simulink model "MPC"  (R2018b)
settings: Solver=VariableStepAuto  StartTime=0.0  StopTime=5  RelTol=1e-3
libraries: mpclib x2
settings Model: Creator=dongdaming  LastModifiedBy=dongdaming

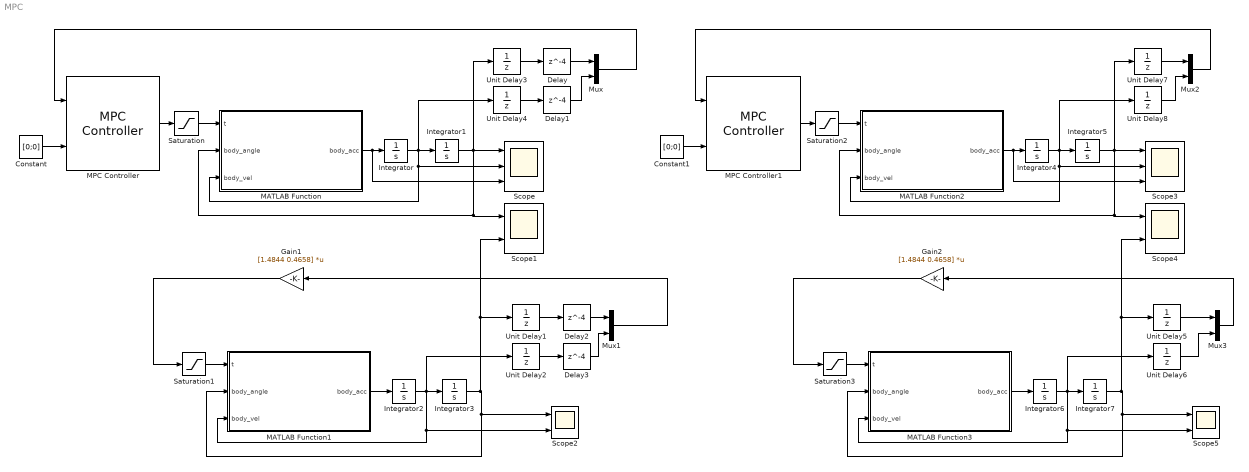
== system MPC ==
  Constant : Constant  Value=[0;0]
  Constant1 : Constant  Value=[0;0]
  Delay{,1..3} (4 alike) : Delay  DelayLength=4
  Gain1 : Gain  Gain=[1.4844 0.4658]  Multiplication=Matrix(K*u)
  Gain2 : Gain  Gain=[1.4844 0.4658]  Multiplication=Matrix(K*u)
  Integrator{,2,4,6} (4 alike) : Integrator
  Integrator1 : Integrator  InitialCondition=pi/3  UpperSaturationLimit=pi  LowerSaturationLimit=-pi
  Integrator3 : Integrator  InitialCondition=pi/3  LimitOutput=on  UpperSaturationLimit=pi  LowerSaturationLimit=-pi
  Integrator5 : Integrator  InitialCondition=pi/3  UpperSaturationLimit=pi  LowerSaturationLimit=-pi
  Integrator7 : Integrator  InitialCondition=pi/3  LimitOutput=on  UpperSaturationLimit=pi  LowerSaturationLimit=-pi
  MATLAB Function : MATLAB Function  TreatAsAtomicUnit=on
  MATLAB Function1 : MATLAB Function  TreatAsAtomicUnit=on
  MATLAB Function2 : MATLAB Function  TreatAsAtomicUnit=on
  MATLAB Function3 : MATLAB Function  TreatAsAtomicUnit=on
  MPC Controller : mpclib/MPC Controller  SCDEnableBlockLinearizationSpecification=on  mpcobj=mpc1  is_multiple=0  enable_value=0  return_u0=off  updateMPCinCallerWorkspace=on  md_inport=off  mv_inport=off  return_cost=off  return_mvseq=off  return_qpstatus=off  return_xseq=off  return_state=off  return_ovseq=off  state_inport=off  umin_inport=off  umax_inport=off  ymin_inport=off  ymax_inport=off  cc_inport=off  ywt_inport=off  uwt_inport=off  duwt_inport=off  rhoeps_inport=off  uref_inport=off  n_ts=0.002  n_p=20  n_mv=1  n_md=0  n_ud=0  n_mo=2  n_uo=0  BlockDataType=double  SampleTimeInherited=off  switch_inport=off
  MPC Controller1 : mpclib/MPC Controller  SCDEnableBlockLinearizationSpecification=on  mpcobj=mpc1  is_multiple=0  enable_value=0  return_u0=off  updateMPCinCallerWorkspace=on  md_inport=off  mv_inport=off  return_cost=off  return_mvseq=off  return_qpstatus=off  return_xseq=off  return_state=off  return_ovseq=off  state_inport=off  umin_inport=off  umax_inport=off  ymin_inport=off  ymax_inport=off  cc_inport=off  ywt_inport=off  uwt_inport=off  duwt_inport=off  rhoeps_inport=off  uref_inport=off  n_ts=0.002  n_p=20  n_mv=1  n_md=0  n_ud=0  n_mo=2  n_uo=0  BlockDataType=double  SampleTimeInherited=off  switch_inport=off
  Mux{,1..3} (4 alike) : Mux  Inputs=2
  Saturation{,1..3} (4 alike) : Saturate  UpperLimit=1.4  LowerLimit=-1.4
  Scope : Scope  NumInputPorts=3
  Scope{1..2,4..5} (4 alike) : Scope  NumInputPorts=2
  Scope3 : Scope  NumInputPorts=3
  Unit Delay{1,3,5,7} (4 alike) : UnitDelay  SampleTime=0.002
  Unit Delay{2,4,6,8} (4 alike) : UnitDelay  InitialCondition=pi/3  SampleTime=0.002
  wires:
  Integrator/1 -> Unit Delay4/1, MATLAB Function/3(body_vel), Scope/2, Integrator1/1
  Integrator1/1 -> Unit Delay3/1, Scope1/1, MATLAB Function/2(body_angle), Scope/1
  Constant/1 -> MPC Controller/2
  Mux/1 -> MPC Controller/1
  MATLAB Function/1(body_acc) -> Scope/3, Integrator/1
  Saturation/1 -> MATLAB Function/1(t)
  MPC Controller/1 -> Saturation/1
  Saturation1/1 -> MATLAB Function1/1(t)
  MATLAB Function1/1(body_acc) -> Integrator2/1
  Integrator3/1 -> Scope1/2, Unit Delay1/1, MATLAB Function1/2(body_angle), Scope2/1
  Integrator2/1 -> Unit Delay2/1, Integrator3/1, Scope2/2, MATLAB Function1/3(body_vel)
  Gain1/1 -> Saturation1/1
  Mux1/1 -> Gain1/1
  Unit Delay3/1 -> Delay/1
  Delay/1 -> Mux/1
  Unit Delay4/1 -> Delay1/1
  Delay1/1 -> Mux/2
  Unit Delay1/1 -> Delay2/1
  Delay2/1 -> Mux1/1
  Unit Delay2/1 -> Delay3/1
  Delay3/1 -> Mux1/2
  Unit Delay6/1 -> Mux3/2
  Unit Delay5/1 -> Mux3/1
  Unit Delay8/1 -> Mux2/2
  Unit Delay7/1 -> Mux2/1
  Mux3/1 -> Gain2/1
  Gain2/1 -> Saturation3/1
  Integrator6/1 -> MATLAB Function3/3(body_vel), Scope5/2, Integrator7/1, Unit Delay6/1
  Integrator7/1 -> Scope5/1, MATLAB Function3/2(body_angle), Unit Delay5/1, Scope4/2
  MATLAB Function3/1(body_acc) -> Integrator6/1
  Saturation3/1 -> MATLAB Function3/1(t)
  MPC Controller1/1 -> Saturation2/1
  Saturation2/1 -> MATLAB Function2/1(t)
  MATLAB Function2/1(body_acc) -> Integrator4/1, Scope3/3
  Mux2/1 -> MPC Controller1/1
  Constant1/1 -> MPC Controller1/2
  Integrator5/1 -> Scope3/1, MATLAB Function2/2(body_angle), Scope4/1, Unit Delay7/1
  Integrator4/1 -> Integrator5/1, Scope3/2, MATLAB Function2/3(body_vel), Unit Delay8/1

== matlab function MPC/MATLAB Function1 ==
  data: t input; body_acc output; body_angle input; body_vel input
function body_acc = fcn(t,body_angle,body_vel)
body_acc=(+1429.48*sin(body_angle)-1215.55*t-2083.85*t*cos(body_angle)-3.87597*sin(2*body_angle)*body_vel^2)/(2.91931+cos(body_angle)^2+8.75194*sin(body_angle)^2);

== matlab function MPC/MATLAB Function ==
  data: t input; body_acc output; body_angle input; body_vel input
function body_acc = fcn(t,body_angle,body_vel)
body_acc=(+1429.48*sin(body_angle)-1215.55*t-2083.85*t*cos(body_angle)-3.87597*sin(2*body_angle)*body_vel^2)/(2.91931+cos(body_angle)^2+8.75194*sin(body_angle)^2);

== matlab function MPC/MATLAB Function2 ==
  data: t input; body_acc output; body_angle input; body_vel input
function body_acc = fcn(t,body_angle,body_vel)
body_acc=(+1429.48*sin(body_angle)-1215.55*t-2083.85*t*cos(body_angle)-3.87597*sin(2*body_angle)*body_vel^2)/(2.91931+cos(body_angle)^2+8.75194*sin(body_angle)^2);

== matlab function MPC/MATLAB Function3 ==
  data: t input; body_acc output; body_angle input; body_vel input
function body_acc = fcn(t,body_angle,body_vel)
body_acc=(+1429.48*sin(body_angle)-1215.55*t-2083.85*t*cos(body_angle)-3.87597*sin(2*body_angle)*body_vel^2)/(2.91931+cos(body_angle)^2+8.75194*sin(body_angle)^2);
